simulink model "Ejercicio2"  (R2023b)
settings: Solver=VariableStepAuto  StartTime=0.0  StopTime=10.0  RelTol=1e-3
undefined symbols (not defined in the file): K, sys2
settings Model: Creator=lopez  LastModifiedBy=lopez

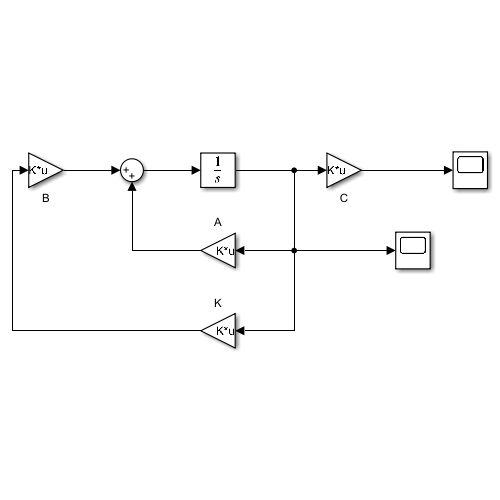
[thumbnail: Simulink's stored preview of the top-level diagram]
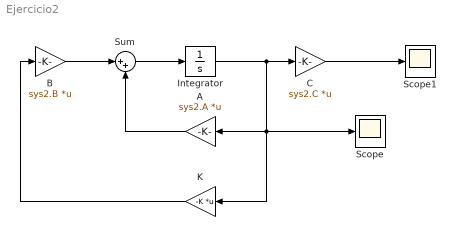
== system Ejercicio2 ==
  A : Gain  Gain=sys2.A  Multiplication=Matrix(K*u)
  B : Gain  Gain=sys2.B  Multiplication=Matrix(K*u)
  C : Gain  Gain=sys2.C  Multiplication=Matrix(K*u)
  Integrator : Integrator
  K : Gain  Gain=-K  Multiplication=Matrix(K*u)
  Scope : Scope
  Scope1 : Scope
  Sum : Sum  Inputs=|++
  wires:
  B/1 -> Sum/1
  Sum/1 -> Integrator/1
  Integrator/1 -> Scope/1, K/1, A/1, C/1
  C/1 -> Scope1/1
  A/1 -> Sum/2
  K/1 -> B/1
